simulink model "Pacemaker_Final"  (R2020a)
settings: Solver=FixedStepAuto  StartTime=0.0  StopTime=Inf  FixedStep=1e-3  RelTol=1e-3
undefined symbols (not defined in the file): D0, D1, D10, D11, D12, D13, D2, D3, D4, D5, D6, D7, D8, D9, PTA0, PTA1, PTA2, PTB23, PTB9, PTC16, PTC17, PTC2, PTC3, PTC4, PTD0, PTD1, PTD2, PTD3
libraries: frdmk64flib x18, simulink x15
settings Model: ExtModeTrigDuration=5  Creator=aryan  LastModifiedBy=Daniel
settings OptimizationCC: EnhancedBackFolding=on  PassReuseOutputArgsAs=Individual arguments  ZeroExternalMemoryAtStartup=off  ZeroInternalMemoryAtStartup=off  MaxStackSize=64  OptimizeBlockOrder=speed  DifferentSizesBufferReuse=on  OptimizationCustomize=off  EfficientTunableParamExpr=on
settings DebuggingCC: ParameterTunabilityLossMsg=error
settings HardwareCC: ProdBitPerPointer=32  ProdBitPerSizeT=32  ProdBitPerPtrDiffT=32  ProdLargestAtomicInteger=Long  ProdLargestAtomicFloat=Double  ProdWordSize=32  ProdHWDeviceType=ARM Compatible->ARM Cortex
settings SFSimCC: MATLABDynamicMemAlloc=off
settings RTWCC: SystemTargetFile=ert.tlc  HardwareBoard=NXP FRDM-K64F  TemplateMakefile=ert_default_tmf  Toolchain=GNU Tools for ARM Embedded Processors
settings CodeAppCC: ForceParamTrailComments=on  IgnoreCustomStorageClasses=off  OperatorAnnotations=on  SimulinkDataObjDesc=on  SFDataObjDesc=on  InsertBlockDesc=on
settings ERTTargetCC: SupportContinuousTime=on  ExtModeTransport=4  ExtModeMexFile=sendToCommService

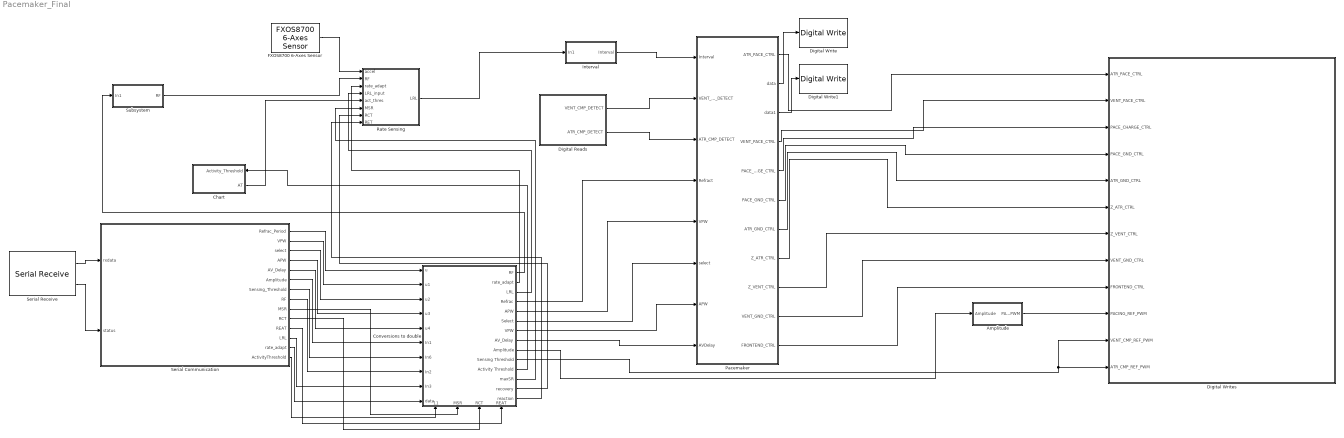
== system Pacemaker_Final ==
  Amplitude : Subsystem
  Chart : Stateflow chart  TreatAsAtomicUnit=on
      settings: PortSchema="{\"entries\":[{\"content\":{\"sides\":[{\"content\":{\"connectorIds\":[]},\"type\":\"ConnectorPlacement.EquallySpacedRectSide\",\"uuid\":\"42c5a6a8-69c1-41b5-99c8-1390670a4b47\"},{\"content\":{\"connectorIds\":[\"In1\",\"Out1\"],\"side\":\"RIGHT\"},\"type\":\"ConnectorPlacement.EquallySpacedRectSide\",\"uuid\":\"944f96d4-89ad-40bf-93b7-42c8f8697fa2\"},{\"content\":{\"connectorIds\":[],\"side\":\"TOP\"},\"type\":\"ConnectorPlacement.EquallySpacedRectSide\",\"uuid\":\"6c0a3315-bf58-494e-a025-9a9813242d09\"}]},\"type\":\"ConnectorPlacement.EquallySpacedConnector\",\"uuid\":\"a3111f38-5aea-48a5-b1ab-4e5ccaec3e7b\"}],\"packageUris\":[\"http://schema.mathworks.com/mf0/Connector/19700101\"],\"version\":\"1.0\"}"
  Conversions to double : Subsystem
      settings: PortSchema="{\"entries\":[{\"content\":{\"sides\":[{\"content\":{\"connectorIds\":[\"In1\",\"In2\",\"In3\",\"In4\",\"In5\",\"In6\",\"In7\",\"In8\",\"In9\",\"In10\"]},\"type\":\"ConnectorPlacement.EquallySpacedRectSide\",\"uuid\":\"4d24861a-2112-40d5-a0e7-6eb08bd24e17\"},{\"content\":{\"connectorIds\":[\"Out1\",\"Out2\",\"Out3\",\"Out4\",\"Out5\",\"Out6\",\"Out7\",\"Out8\",\"Out9\",\"Out10\",\"Out11\",\"Out12\",\"Out13\",\"Out14\"],\"side\":\"RIGHT\"},\"type\":\"ConnectorPlacement.EquallySpacedRectSide\",\"uuid\":\"efac6499-c383-4404-918d-e6a23ac4b892\"},{\"content\":{\"connectorIds\":[],\"side\":\"TOP\"},\"type\":\"ConnectorPlacement.EquallySpacedRectSide\",\"uuid\":\"a8df73dc-f2de-445c-9663-e5a665afcd05\"},{\"content\":{\"connectorIds\":[\"In11\",\"In12\",\"In13\",\"In14\"],\"side\":\"BOTTOM\"},\"type\":\"ConnectorPlacement.EquallySpacedRectSide\",\"uuid\":\"7d4ccbea-e744-45e2-85a4-e75bcb924ee4\"}]},\"type\":\"ConnectorPlacement.EquallySpacedConnector\",\"uuid\":\"0b6d23ad-f8c4-4562-98cc-50cfb679a7c2\"}],\"packageUris\":[\"http://schema.mathworks.com/mf0/Connector/19700101\"],\"version\":\"1.0\"}"
  Digital Reads : Subsystem
  Digital Write : frdmk64flib/Digital Write  Whichpin=RED_LED
  Digital Write1 : frdmk64flib/Digital Write  Whichpin=GREEN_LED
  Digital Writes : Subsystem
  FXOS8700 6-Axes Sensor : frdmk64flib/FXOS8700 6-Axes Sensor  Activesensor=Accelerometer only  ODR=800Hz  HybridODR=400Hz  Accelfullrange=-2g to +2g  SampleTime=-1
  Interval : Subsystem
  Pacemaker : Stateflow chart  TreatAsAtomicUnit=on
      settings: PortSchema="{\"entries\":[{\"content\":{\"sides\":[{\"content\":{\"connectorIds\":[\"In1\",\"In2\",\"In8\",\"In3\",\"In4\",\"In5\",\"In6\",\"In7\"]},\"type\":\"ConnectorPlacement.EquallySpacedRectSide\",\"uuid\":\"48e8cfa6-1b63-4154-ae39-d83175eff6b5\"},{\"content\":{\"connectorIds\":[\"Out1\",\"Out2\",\"Out3\",\"Out4\",\"Out5\",\"Out6\",\"Out7\",\"Out8\",\"Out9\",\"Out10\",\"Out11\"],\"side\":\"RIGHT\"},\"type\":\"ConnectorPlacement.EquallySpacedRectSide\",\"uuid\":\"2c49f9e8-e17d-477a-ac75-d4910fa58ffc\"},{\"content\":{\"connectorIds\":[],\"side\":\"TOP\"},\"type\":\"ConnectorPlacement.EquallySpacedRectSide\",\"uuid\":\"8b4e7d54-eec3-43a6-9cbf-8ef4b56e1046\"}]},\"type\":\"ConnectorPlacement.EquallySpacedConnector\",\"uuid\":\"611e33bb-eecb-417e-81e9-efd076cd5135\"}],\"packageUris\":[\"http://schema.mathworks.com/mf0/Connector/19700101\"],\"version\":\"1.0\"}"
  Rate Sensing : Stateflow chart  TreatAsAtomicUnit=on
  Serial Communication : Stateflow chart  TreatAsAtomicUnit=on
      settings: PortSchema="{\"entries\":[{\"content\":{\"sides\":[{\"content\":{\"connectorIds\":[\"In1\",\"In2\"]},\"type\":\"ConnectorPlacement.EquallySpacedRectSide\",\"uuid\":\"5ab76470-15da-4127-94e5-6eb23ac48143\"},{\"content\":{\"connectorIds\":[\"Out2\",\"Out3\",\"Out4\",\"Out5\",\"Out6\",\"Out7\",\"Out8\",\"Out11\",\"Out12\",\"Out13\",\"Out14\",\"Out1\",\"Out9\",\"Out10\"],\"side\":\"RIGHT\"},\"type\":\"ConnectorPlacement.EquallySpacedRectSide\",\"uuid\":\"8e5b6f80-3e75-4a08-82bd-75b30b4886ca\"},{\"content\":{\"connectorIds\":[],\"side\":\"TOP\"},\"type\":\"ConnectorPlacement.EquallySpacedRectSide\",\"uuid\":\"f4d9c5be-38df-4b86-a579-d3d9d23e8438\"}]},\"type\":\"ConnectorPlacement.EquallySpacedConnector\",\"uuid\":\"427b7b80-35a8-45f5-a0db-c457df1d244e\"}],\"packageUris\":[\"http://schema.mathworks.com/mf0/Connector/19700101\"],\"version\":\"1.0\"}"
  Serial Receive : frdmk64flib/Serial Receive  SCIModule=0  Baudrate=uint32(9600)  Parity=None  StopBits=1  HardwareFlowControl=None  ByteOrder=LittleEndian  DataType=uint8  DataLength=18  BlockingMode=off  OutputStatus=on  SampleTime=-1
  Subsystem : Subsystem
  wires:
  Pacemaker/4(VENT_PACE_CTRL) -> Digital Writes/2(VENT_PACE_CTRL)
  Pacemaker/5(PACE_CHARGE_CTRL) -> Digital Writes/3(PACE_CHARGE_CTRL)
  Pacemaker/1(ATR_PACE_CTRL) -> Digital Writes/1(ATR_PACE_CTRL)
  Pacemaker/8(Z_ATR_CTRL) -> Digital Writes/6(Z_ATR_CTRL)
  Pacemaker/7(ATR_GND_CTRL) -> Digital Writes/5(ATR_GND_CTRL)
  Pacemaker/6(PACE_GND_CTRL) -> Digital Writes/4(PACE_GND_CTRL)
  Digital Reads/1(VENT_CMP_DETECT) -> Pacemaker/2(VENT_CMP_DETECT)
  Pacemaker/11(FRONTEND_CTRL) -> Digital Writes/9(FRONTEND_CTRL)
  Pacemaker/9(Z_VENT_CTRL) -> Digital Writes/7(Z_VENT_CTRL)
  Pacemaker/10(VENT_GND_CTRL) -> Digital Writes/8(VENT_GND_CTRL)
  Interval/1(Interval) -> Pacemaker/1(Interval)
  Amplitude/1(PACING_REF_PWM) -> Digital Writes/10(PACING_REF_PWM)
  Digital Reads/2(ATR_CMP_DETECT) -> Pacemaker/8(ATR_CMP_DETECT)
  FXOS8700 6-Axes Sensor/1 -> Rate Sensing/1(accel)
  Subsystem/1(RF) -> Rate Sensing/2(RF)
  Serial Receive/2 -> Serial Communication/2(status)
  Serial Receive/1 -> Serial Communication/1(rxdata)
  Serial Communication/2(Refrac_Period) -> Conversions to double/1(u)
  Serial Communication/3(VPW) -> Conversions to double/2(u1)
  Serial Communication/5(APW) -> Conversions to double/4(u3)
  Serial Communication/6(AV_Delay) -> Conversions to double/5(u4)
  Serial Communication/4(select) -> Conversions to double/3(u2)
  Conversions to double/4(Refrac) -> Pacemaker/3(Refract)
  Conversions to double/5(APW) -> Pacemaker/4(VPW)
  Conversions to double/6(Select) -> Pacemaker/5(select)
  Conversions to double/7(VPW) -> Pacemaker/6(APW)
  Conversions to double/8(AV_Delay) -> Pacemaker/7(AVDelay)
  Serial Communication/7(Amplitude) -> Conversions to double/6(In1)
  Serial Communication/8(Sensing_Threshold) -> Conversions to double/7(In6)
  Conversions to double/10(Sensing Threshold) -> Digital Writes/11(VENT_CMP_REF_PWM), Digital Writes/12(ATR_CMP_REF_PWM)
  Conversions to double/9(Amplitude) -> Amplitude/1(Amplitude)
  Serial Communication/11(RF) -> Conversions to double/8(In2)
  Serial Communication/1(LRL) -> Conversions to double/9(In3)
  Conversions to double/3(LRL) -> Rate Sensing/4(LRL_input)
  Conversions to double/1(RF) -> Subsystem/1(In1)
  Serial Communication/9(rate_adapt) -> Conversions to double/10(data)
  Conversions to double/2(rate_adapt) -> Rate Sensing/3(rate_adapt)
  Serial Communication/10(ActivityThreshold) -> Conversions to double/11(ActivityThreshold)
  Serial Communication/12(MSR) -> Conversions to double/12(MSR)
  Serial Communication/13(RCT) -> Conversions to double/13(RCT)
  Serial Communication/14(REAT) -> Conversions to double/14(REAT)
  Conversions to double/12(maxSR) -> Rate Sensing/6(MSR)
  Conversions to double/13(recovery) -> Rate Sensing/7(RCT)
  Conversions to double/14(reaction) -> Rate Sensing/8(RET)
  Conversions to double/11(Activity Threshold) -> Chart/1(Activity_Threshold)
  Chart/1(AT) -> Rate Sensing/5(act_thres)
  Pacemaker/2(data) -> Digital Write/1
  Rate Sensing/1(LRL) -> Interval/1(In1)
  Pacemaker/3(data1) -> Digital Write1/1

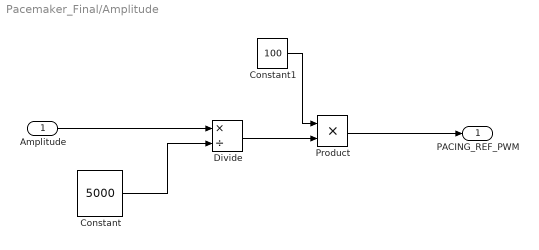
== system Pacemaker_Final/Amplitude ==
  Amplitude : Inport
  Constant : Constant  Value=5000
  Constant1 : Constant  Value=100
  Divide : Product  Inputs=*/
  Product : Product
  PACING_REF_PWM : Outport
  wires:
  Constant/1 -> Divide/2
  Divide/1 -> Product/2
  Constant1/1 -> Product/1
  Product/1 -> PACING_REF_PWM/1
  Amplitude/1 -> Divide/1

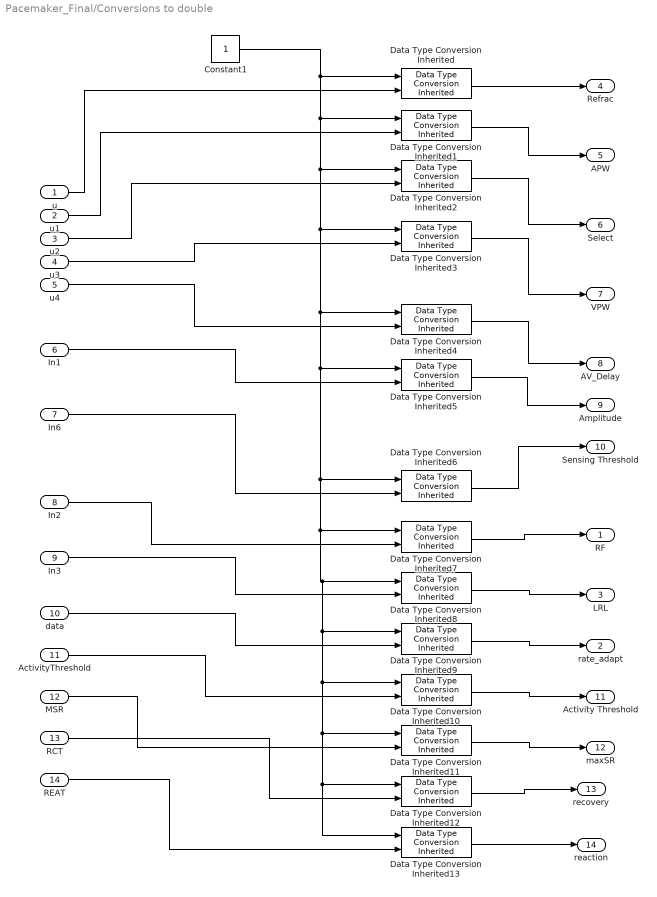
== system Pacemaker_Final/Conversions to double ==
  u : Inport
  u1 : Inport  Port=2
  u2 : Inport  Port=3
  u3 : Inport  Port=4
  u4 : Inport  Port=5
  In1 : Inport  Port=6
  In6 : Inport  Port=7
  In2 : Inport  Port=8
  In3 : Inport  Port=9
  data : Inport  Port=10
  ActivityThreshold : Inport  Port=11
  MSR : Inport  Port=12
  RCT : Inport  Port=13
  REAT : Inport  Port=14
  Constant1 : Constant
  Data Type Conversion Inherited{,1..13} (14 alike) : simulink/Signal Attributes/Data Type Conversion Inherited  ConvertRealWorld=Real World Value  DoSatur=off
      settings: SourceProductBaseCode=SL
  RF : Outport
  rate_adapt : Outport  Port=2
  LRL : Outport  Port=3
  Refrac : Outport  Port=4
  APW : Outport  Port=5
  Select : Outport  Port=6
  VPW : Outport  Port=7
  AV_Delay : Outport  Port=8
  Amplitude : Outport  Port=9
  Sensing Threshold : Outport  Port=10
  Activity Threshold : Outport  Port=11
  maxSR : Outport  Port=12
  recovery : Outport  Port=13
  reaction : Outport  Port=14
  wires:
  Data Type Conversion Inherited4/1 -> AV_Delay/1
  u/1 -> Data Type Conversion Inherited/2
  Data Type Conversion Inherited1/1 -> APW/1
  u2/1 -> Data Type Conversion Inherited2/2
  Data Type Conversion Inherited3/1 -> VPW/1
  u3/1 -> Data Type Conversion Inherited3/2
  u1/1 -> Data Type Conversion Inherited1/2
  u4/1 -> Data Type Conversion Inherited4/2
  Data Type Conversion Inherited2/1 -> Select/1
  Data Type Conversion Inherited/1 -> Refrac/1
  In6/1 -> Data Type Conversion Inherited6/2
  In1/1 -> Data Type Conversion Inherited5/2
  Data Type Conversion Inherited5/1 -> Amplitude/1
  Data Type Conversion Inherited6/1 -> Sensing Threshold/1
  In2/1 -> Data Type Conversion Inherited7/2
  In3/1 -> Data Type Conversion Inherited8/2
  Data Type Conversion Inherited7/1 -> RF/1
  Data Type Conversion Inherited8/1 -> LRL/1
  data/1 -> Data Type Conversion Inherited9/2
  Constant1/1 -> Data Type Conversion Inherited13/1, Data Type Conversion Inherited12/1, Data Type Conversion Inherited11/1, Data Type Conversion Inherited10/1, Data Type Conversion Inherited9/1, Data Type Conversion Inherited8/1, Data Type Conversion Inherited7/1, Data Type Conversion Inherited6/1, Data Type Conversion Inherited5/1, Data Type Conversion Inherited4/1, Data Type Conversion Inherited3/1, Data Type Conversion Inherited2/1, Data Type Conversion Inherited1/1, Data Type Conversion Inherited/1
  Data Type Conversion Inherited9/1 -> rate_adapt/1
  ActivityThreshold/1 -> Data Type Conversion Inherited10/2
  Data Type Conversion Inherited10/1 -> Activity Threshold/1
  MSR/1 -> Data Type Conversion Inherited11/2
  RCT/1 -> Data Type Conversion Inherited12/2
  REAT/1 -> Data Type Conversion Inherited13/2
  Data Type Conversion Inherited11/1 -> maxSR/1
  Data Type Conversion Inherited13/1 -> reaction/1
  Data Type Conversion Inherited12/1 -> recovery/1

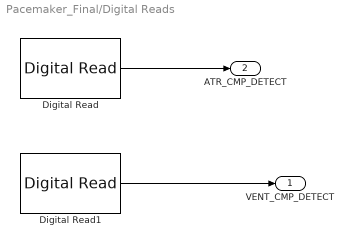
== system Pacemaker_Final/Digital Reads ==
  Digital Read : frdmk64flib/Digital Read  Whichpin=PTC16 (D0)  SampleTime=-1
  Digital Read1 : frdmk64flib/Digital Read  Whichpin=PTC17 (D1)  SampleTime=-1
  VENT_CMP_DETECT : Outport
  ATR_CMP_DETECT : Outport  Port=2
  wires:
  Digital Read1/1 -> VENT_CMP_DETECT/1
  Digital Read/1 -> ATR_CMP_DETECT/1

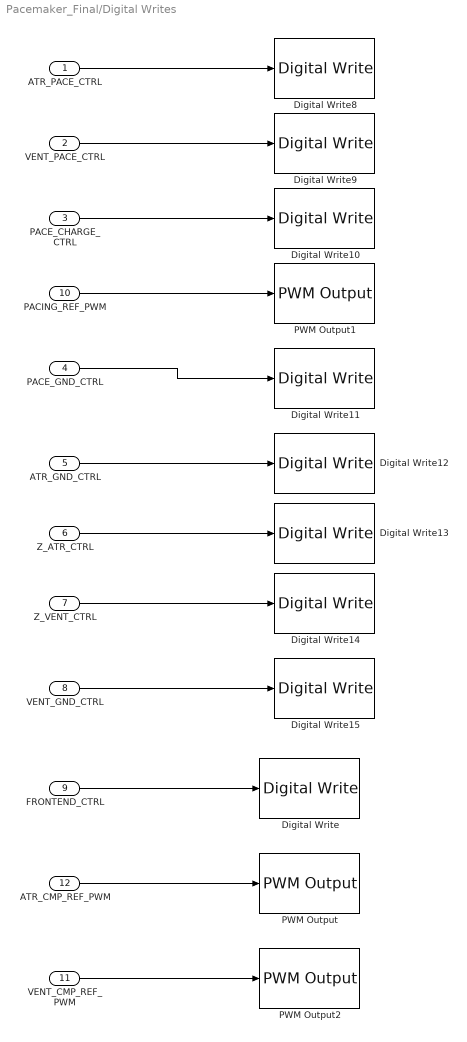
== system Pacemaker_Final/Digital Writes ==
  ATR_PACE_CTRL : Inport
  VENT_PACE_CTRL : Inport  Port=2
  PACE_CHARGE_CTRL : Inport  Port=3
  PACE_GND_CTRL : Inport  Port=4
  ATR_GND_CTRL : Inport  Port=5
  Z_ATR_CTRL : Inport  Port=6
  Z_VENT_CTRL : Inport  Port=7
  VENT_GND_CTRL : Inport  Port=8
  FRONTEND_CTRL : Inport  Port=9
  PACING_REF_PWM : Inport  Port=10
  VENT_CMP_REF_PWM : Inport  Port=11
  ATR_CMP_REF_PWM : Inport  Port=12
  Digital Write : frdmk64flib/Digital Write  Whichpin=PTD1 (D13)
  Digital Write10 : frdmk64flib/Digital Write  Whichpin=PTB9 (D2)
  Digital Write11 : frdmk64flib/Digital Write  Whichpin=PTD0 (D10)
  Digital Write12 : frdmk64flib/Digital Write  Whichpin=PTD2 (D11)
  Digital Write13 : frdmk64flib/Digital Write  Whichpin=PTB23 (D4)
  Digital Write14 : frdmk64flib/Digital Write  Whichpin=PTC3 (D7)
  Digital Write15 : frdmk64flib/Digital Write  Whichpin=PTD3 (D12)
  Digital Write8 : frdmk64flib/Digital Write  Whichpin=PTA0 (D8)
  Digital Write9 : frdmk64flib/Digital Write  Whichpin=PTC4 (D9)
  PWM Output : frdmk64flib/PWM Output  Whichpin=PTC2 (D6)  InitialFrequency=2000  InitialDutyCycle=80
  PWM Output1 : frdmk64flib/PWM Output  Whichpin=PTA2 (D5)  InitialFrequency=2000  InitialDutyCycle=70
  PWM Output2 : frdmk64flib/PWM Output  Whichpin=PTA1 (D3)  InitialFrequency=2000  InitialDutyCycle=80
  wires:
  ATR_PACE_CTRL/1 -> Digital Write8/1
  VENT_PACE_CTRL/1 -> Digital Write9/1
  PACE_CHARGE_CTRL/1 -> Digital Write10/1
  PACING_REF_PWM/1 -> PWM Output1/1
  PACE_GND_CTRL/1 -> Digital Write11/1
  ATR_GND_CTRL/1 -> Digital Write12/1
  Z_ATR_CTRL/1 -> Digital Write13/1
  Z_VENT_CTRL/1 -> Digital Write14/1
  VENT_GND_CTRL/1 -> Digital Write15/1
  FRONTEND_CTRL/1 -> Digital Write/1
  VENT_CMP_REF_PWM/1 -> PWM Output2/1
  ATR_CMP_REF_PWM/1 -> PWM Output/1

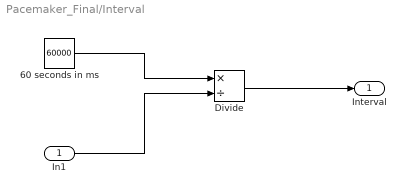
== system Pacemaker_Final/Interval ==
  In1 : Inport
  60 seconds in ms : Constant  Value=60000
  Divide : Product  Inputs=*/
  Interval : Outport
  wires:
  60 seconds in ms/1 -> Divide/1
  In1/1 -> Divide/2
  Divide/1 -> Interval/1

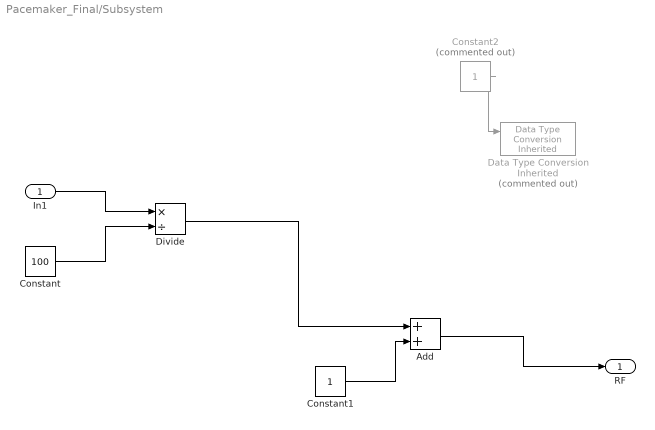
== system Pacemaker_Final/Subsystem ==
  In1 : Inport
  Add : Sum
  Constant : Constant  Value=100  OutDataTypeStr=double
  Constant1 : Constant  OutDataTypeStr=double
  Constant2 : Constant  Commented=on  OutDataTypeStr=double
  Data Type Conversion Inherited : simulink/Signal Attributes/Data Type Conversion Inherited  Commented=on  ConvertRealWorld=Real World Value  DoSatur=off
      settings: SourceProductBaseCode=SL
  Divide : Product  Inputs=*/
  RF : Outport
  wires:
  Constant1/1 -> Add/2
  Constant2/1 -> Data Type Conversion Inherited/1
  In1/1 -> Divide/1
  Constant/1 -> Divide/2
  Divide/1 -> Add/1
  Add/1 -> RF/1

== stateflow chart Pacemaker_Final/Pacemaker ==
  settings: executeAtInitialization=1
  state AOO_Charge_Discharge
    entry:
    data = 0;
    FRONTEND_CTRL = false;
    PACE_GND_CTRL = true;
    ATR_PACE_CTRL = false;
    VENT_PACE_CTRL = false;
    ATR_GND_CTRL = true;
    VENT_GND_CTRL = false;
    Z_ATR_CTRL = false;
    Z_VENT_CTRL = false;
    PACE_CHARGE_CTRL = true;
  state AOO_Pacing
    entry:
    data = 1;
    PACE_CHARGE_CTRL = false;
    ATR_GND_CTRL = false;
    ATR_PACE_CTRL = true;
  state VOO_Pacing
    entry:
    data1 = 1;
    PACE_CHARGE_CTRL = false;
    VENT_GND_CTRL = false;
    VENT_PACE_CTRL = true;
  state VOO_Charge_Discharge
    entry:
    data1 = 0;
    FRONTEND_CTRL = false;
    PACE_GND_CTRL = true;
    ATR_PACE_CTRL = false;
    VENT_PACE_CTRL = false;
    ATR_GND_CTRL = false;
    VENT_GND_CTRL = true;
    Z_ATR_CTRL = false;
    Z_VENT_CTRL = false;
    PACE_CHARGE_CTRL = true;
  state AAI_Charge_Discharge
    entry:
    data = 0;
    FRONTEND_CTRL = true;
    PACE_GND_CTRL = true;
    ATR_PACE_CTRL = false;
    VENT_PACE_CTRL = false;
    ATR_GND_CTRL = true;
    VENT_GND_CTRL = false;
    Z_ATR_CTRL = false;
    Z_VENT_CTRL = false;
    PACE_CHARGE_CTRL = true;
  state AAI_Pacing
    entry:
    data = 1;
    PACE_CHARGE_CTRL = false;
    ATR_GND_CTRL = false;
    ATR_PACE_CTRL = true;
  state Mode_Select
  state VVI_Charge_Discharge
    entry:
    data1 = 0;
    FRONTEND_CTRL = true;
    PACE_GND_CTRL = true;
    ATR_PACE_CTRL = false;
    VENT_PACE_CTRL = false;
    ATR_GND_CTRL = false;
    VENT_GND_CTRL = true;
    Z_ATR_CTRL = false;
    Z_VENT_CTRL = false;
    PACE_CHARGE_CTRL = true;
  state VVI_Pacing
    entry:
    data1 = 1;
    PACE_CHARGE_CTRL = false;
    VENT_GND_CTRL = false;
    VENT_PACE_CTRL = true;
  state V_Pace
    entry:
    data1 = 1;
    PACE_CHARGE_CTRL=false;
    PACE_GND_CTRL=true;
    ATR_PACE_CTRL=false;
    ATR_GND_CTRL=false;
    Z_ATR_CTRL=false;
    Z_VENT_CTRL=false;
    VENT_GND_CTRL=false;
    VENT_PACE_CTRL=true;
  state DOO
    entry:
    data1 = 0;
    FRONTEND_CTRL = false;
    ATR_PACE_CTRL=false;
    VENT_PACE_CTRL=false;
    PACE_CHARGE_CTRL =true;
    PACE_GND_CTRL=true;
    Z_ATR_CTRL=false;
    Z_VENT_CTRL=false;
    ATR_GND_CTRL=false;
    VENT_GND_CTRL=true;
  state A_Pace
    entry:
    data = 1;
    PACE_CHARGE_CTRL=false;
    PACE_GND_CTRL=true;
    ATR_PACE_CTRL=true;
    ATR_GND_CTRL=false;
    Z_ATR_CTRL=false;
    Z_VENT_CTRL=false;
    VENT_GND_CTRL=false;
    VENT_PACE_CTRL=false;
  state AV_Delay
    entry:
    data = 0;
    FRONTEND_CTRL = false;
    ATR_PACE_CTRL=false;
    VENT_PACE_CTRL=false;
    PACE_CHARGE_CTRL =true;
    PACE_GND_CTRL=true;
    Z_ATR_CTRL=false;
    Z_VENT_CTRL=false;
    ATR_GND_CTRL=true;
    VENT_GND_CTRL=false;
  note: DOO
  AOO_Charge_Discharge -> Mode_Select [order 1] : [select ~= 1]
  AOO_Charge_Discharge -> AOO_Pacing [order 2] : after(Interval-APW,msec)
  AOO_Pacing -> AOO_Charge_Discharge : after(APW,msec)
  Mode_Select -> AOO_Charge_Discharge [order 1] : [select==1]
  VOO_Charge_Discharge -> VOO_Pacing [order 2] : after(Interval-VPW,msec)
  Mode_Select -> VOO_Charge_Discharge [order 4] : [select==2]
  VOO_Pacing -> VOO_Charge_Discharge : after(VPW, msec)
  VOO_Charge_Discharge -> Mode_Select [order 1] : [select ~= 2]
  AAI_Charge_Discharge -> AAI_Charge_Discharge [order 3] : [ATR_CMP_DETECT && after(Refract,msec)]
  AAI_Charge_Discharge -> AAI_Pacing [order 2] : after(Interval-APW,msec)
  (default) -> Mode_Select
  AAI_Pacing -> AAI_Charge_Discharge : after(APW,msec)
  Mode_Select -> AAI_Charge_Discharge [order 5] : [select==3]
  AAI_Charge_Discharge -> Mode_Select [order 1] : [select ~= 3]
  VVI_Charge_Discharge -> Mode_Select [order 1] : [select ~= 4]
  Mode_Select -> VVI_Charge_Discharge [order 2] : [select==4]
  Mode_Select -> DOO [order 3] : [select==5]
  DOO -> Mode_Select [order 1] : [select ~= 5]
  VVI_Charge_Discharge -> VVI_Charge_Discharge [order 3] : [VENT_CMP_DETECT && after(Refract,msec)]
  VVI_Charge_Discharge -> VVI_Pacing [order 2] : after(Interval-VPW,msec)
  VVI_Pacing -> VVI_Charge_Discharge : after(VPW, msec)
  DOO -> A_Pace [order 2] : after(Interval-AVDelay-VPW,msec)
  A_Pace -> AV_Delay : after(APW,msec)
  AV_Delay -> V_Pace : after(AVDelay-APW,msec)
  V_Pace -> DOO : after(VPW,msec)
  data: Interval input; ATR_PACE_CTRL output boolean; data output; data1 output; VENT_PACE_CTRL output boolean; PACE_CHARGE_CTRL output boolean; PACE_GND_CTRL output boolean; ATR_GND_CTRL output boolean; Z_ATR_CTRL output boolean; Z_VENT_CTRL output boolean; VENT_GND_CTRL output boolean; VENT_CMP_DETECT input boolean; Refract input; VPW input; FRONTEND_CTRL output boolean; select input; APW input; AVDelay input; ATR_CMP_DETECT input boolean

== stateflow chart Pacemaker_Final/Serial Communication ==
  settings: executeAtInitialization=1
  state INITIAL
    entry:
    select = 1;
    LRL = 60;
    Refrac_Period = 200;
    AV_Delay = 100;
    APW = 1;
    VPW = 1;
    Amplitude = 4000;
    Sensing_Threshold = 80;
    ActivityThreshold = 1;
    RF = 10;
    rate_adapt = 0;
  state STANDBY
  state READ_PARAMS
    entry:
    select = rxdata(2); %AOO=1, VOO=2, AAI=3, VVI=4, DOO=5
    LRL = rxdata(3);
    Refrac_Period = typecast(rxdata(4:5),'uint16');
    AV_Delay = typecast(rxdata(6:7),'uint16');
    APW = rxdata(8);
    VPW = rxdata(9);
    Amplitude = typecast(rxdata(10:11),'uint16')
    Sensing_Threshold = rxdata(12);
    ActivityThreshold = rxdata(13); %1-7
    RF = rxdata(14); %1-16
    rate_adapt = rxdata(15); % 0 = constant rate, 1 = rate adaptive
    MSR = rxdata(16); %50-175
    RCT = rxdata(17); %2-16
    REAT = rxdata(18); %10-50
  (default) -> INITIAL
  INITIAL -> STANDBY
  STANDBY -> (junction 39) : [status == 0]
  (junction 39) -> READ_PARAMS [order 1] : [rxdata(1) == hex2dec('16')]
  (junction 39) -> STANDBY [order 2]
  READ_PARAMS -> STANDBY
  data: LRL output uint8; Refrac_Period output uint16; VPW output uint8; select output uint8; APW output uint8; AV_Delay output uint16; rxdata input uint8; status input uint8; Amplitude output uint16; Sensing_Threshold output uint8; rate_adapt output uint8; ActivityThreshold output uint8; RF output uint8; MSR output uint8; RCT output uint8; REAT output uint8

== stateflow chart Pacemaker_Final/Rate Sensing ==
  note: Rate Sensing Stateflow
  state Intial
    entry:
    LRL = LRL_input;
  state Reaction
    entry:
    interval = (RET)/(1+(RF-1)*100);
    LRL = LRL + (max(accel))*((RF-1)*100);
    if(LRL >= MSR)
    LRL = MSR;
    end
  state Recovery
    entry:
    bps_dec = (MSR-LRL_input)/RCT/60;
    interval = (RCT*60)/(16+(RF-1)*100);
    LRL = LRL - bps_dec*interval;
  (default) -> Intial
  Intial -> Reaction [order 1] : [ abs(accel(1)) > act_thres || abs(accel(2)) > act_thres || abs(accel(3)) > (1+act_thres) && rate_adapt == 1]
  Reaction -> Reaction [order 2] : after(interval,sec)
  Intial -> Intial [order 2] : [rate_adapt == 0]
  Reaction -> Recovery [order 1] : [ abs(accel(1)) < act_thres && abs(accel(2)) < act_thres && abs(accel(3)) < (1 + act_thres) ]
  Recovery -> Reaction [order 3] : [ abs(accel(1)) >= act_thres && abs(accel(2)) >= act_thres && abs(accel(3)) >=(1+act_thres) ]
  Recovery -> Intial [order 1] : [LRL<=LRL_input]
  Recovery -> Recovery [order 2] : after(interval,sec)
  data: accel input double; LRL output double; RF input double; rate_adapt input double; LRL_input input; act_thres input double; interval local double; bps_dec local double; MSR input double; RCT input double; RET input double

== stateflow chart Pacemaker_Final/Chart ==
  state V_Low
    entry:
    AT = 0.3;
  state Low
    entry:
    AT = 0.5;
  state Low_Med
    entry:
    AT=0.8;
  state Setting
    entry:
  state Med
    entry:
    AT = 1;
  state Med_High
    entry:
    AT = 1.1;
  state High
    entry:
    AT = 1.3;
  state V_High
    entry:
    AT = 1.5;
  Setting -> V_Low [order 1] : [Activity_Threshold == 1]
  Setting -> Low [order 2] : [Activity_Threshold == 2]
  (default) -> Setting
  Setting -> Low_Med [order 3] : [Activity_Threshold == 3]
  Setting -> Med [order 4] : [Activity_Threshold == 4]
  Setting -> Med_High [order 5] : [Activity_Threshold == 5]
  Setting -> High [order 6] : [Activity_Threshold == 6]
  Setting -> V_High [order 7] : [Activity_Threshold == 7]
  data: Activity_Threshold input double; AT output double
